simulink model "Maglev_Hardware_25a_R1"  (R2025a)
settings: Solver=FixedStepDiscrete  StartTime=0.0  StopTime=inf  FixedStep=Ts  RelTol=1e-3  EnableMultiTasking=on
values from neighbouring files (symbols this model uses):
  k = 2.9626e-4    (= 0.00029626)    [rhs.m]    (also in simulate.m = -162.15)
undefined symbols (not defined in the file or in its folder): dend, dspblkCoreblockFVToolHelper, gcbh, numd
libraries: arduinolib x6, simulink x1
settings Model: ModifiedByFormat=C. Gokcek  SimulationMode=external  SILPILModeSetting=veronly  ExtModeTrigDuration=2  Creator=C. Gokcek  LastModifiedBy=C. Gokcek
settings SolverCC: AlgebraicLoopSolver=TrustRegion
settings DataIOCC: LimitDataPoints=on  SaveFormat=Array  SaveOutput=off  SaveTime=off  ReturnWorkspaceOutputs=off
settings OptimizationCC: EnhancedBackFolding=on  PassReuseOutputArgsThreshold=0.0  MaxStackSize=64  OptimizeBlockOrder=speed  DifferentSizesBufferReuse=on  OptimizationCustomize=off
settings DebuggingCC: UnderspecifiedInitializationDetection=Classic  MergeDetectMultiDrivingBlocksExec=none  ParameterTunabilityLossMsg=error  UnconnectedInputMsg=warning  UnconnectedOutputMsg=warning  UnconnectedLineMsg=warning  StateNameClashWarn=warning  SFUnexpectedBacktrackingDiag=warning  SFNoUnconditionalDefaultTransitionDiag=warning  SFExecutionAtInitializationDiag=none  ArithmeticOperatorsInVariantConditions=warning
settings HardwareCC: ProdBitPerInt=16.0  ProdBitPerPointer=16.0  ProdBitPerSizeT=16.0  ProdBitPerPtrDiffT=16.0  ProdLargestAtomicFloat=None  ProdWordSize=8.0  ProdHWDeviceType=Atmel->AVR  UseEmbeddedCoderFeatures=off  UseSimulinkCoderFeatures=off
settings ModelReferenceCC: EnableRefExpFcnMdlSchedulingChecks=on  PropagateSignalLabelsOutOfModel=off
settings SFSimCC: SimUseLocalCustomCode=off  MATLABDynamicMemAlloc=off  CustomCodeUndefinedFunction=UseInterfaceOnly
settings RTWCC: SystemTargetFile=ert.tlc  HardwareBoard=Arduino Mega 2560  TemplateMakefile=ert_default_tmf  RTWVerbose=off  RTWUseLocalCustomCode=off  Toolchain=Arduino AVR  BuildConfiguration=Faster Runs  GPUComputeCapability=3.5  Description=Embedded Coder
settings CodeAppCC: ForceParamTrailComments=on  OperatorAnnotations=on  MangleLength=10.0
settings ERTTargetCC: ExtModeTransport=3.0  ExtModeStaticAllocSize=2048.0  InlinedParameterPlacement=Hierarchical  DynamicArrayContainerType=coder::array  ERTCustomFileBanners=off  SupportContinuousTime=on  SupportNonInlinedSFcns=on  RemoveResetFunc=off  SupportVariableSizeSignals=on  ModelStepFunctionPrototypeControlCompliant=off
settings ConfigComp: CovMetricSettings=dw  CovSaveCumulativeToWorkspaceVar=on  CovSaveSingleToWorkspaceVar=on  CovExternalEMLEnable=off

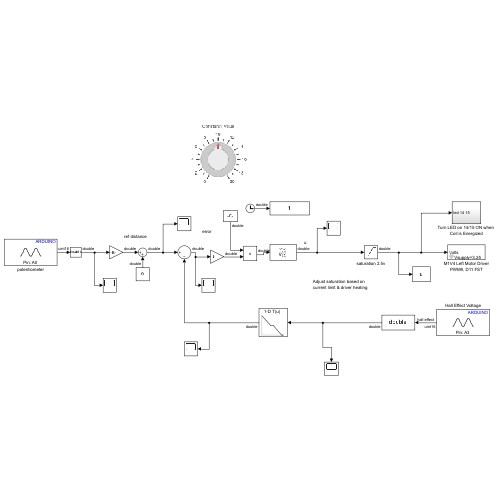
[thumbnail: Simulink's stored preview of the top-level diagram]
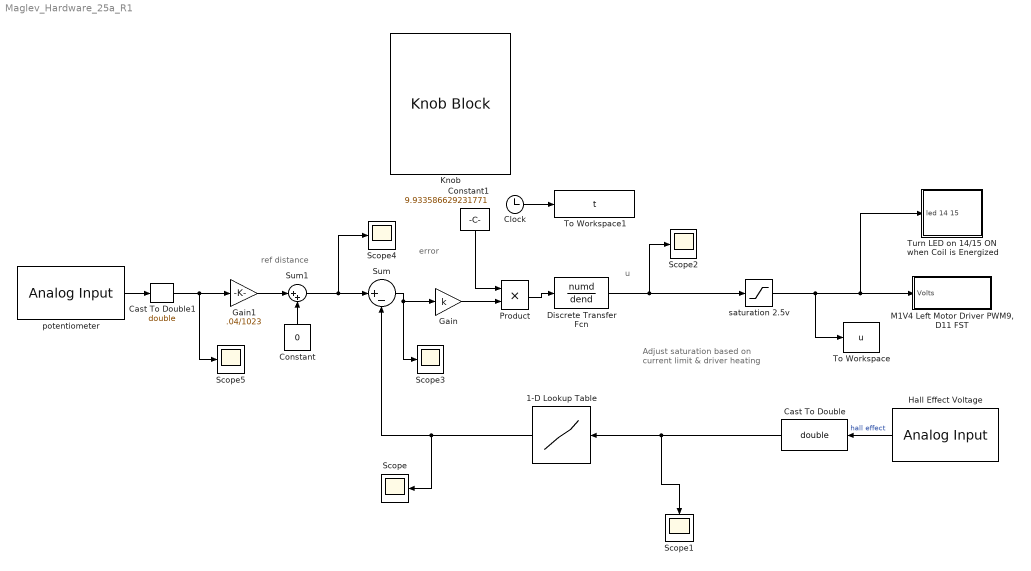
== system Maglev_Hardware_25a_R1 ==
  note: u
  note: error
  note: ref distance
  note: Adjust saturation based on
      | current limit & driver heating
  1-D Lookup Table : Lookup_n-D  NumberOfTableDimensions=1  BreakpointsForDimension1=[530;560;590;610;671;675;680;683]  Table=[0.038;0.034;0.03;0.03;0.022;0.022;0.022;0.022]  InternalRulePriority=Speed  RndMeth=Simplest
  Cast To Double : DataTypeConversion  OutDataTypeStr=double  SaturateOnIntegerOverflow=off  RndMeth=Floor
  Cast To Double1 : DataTypeConversion  OutDataTypeStr=double  SaturateOnIntegerOverflow=off  RndMeth=Floor
  Clock : Clock
  Constant : Constant  Value=0
  Constant1 : Constant  Value=9.933586629231771
  Discrete Transfer Fcn : DiscreteTransferFcn  LoadFcn=dspblkCoreblockFVToolHelper(gcbh,'load');  Numerator=numd  Denominator=dend
      settings: CopyFcn=dspblkCoreblockFVToolHelper(gcbh,'copy');  DeleteFcn=dspblkCoreblockFVToolHelper(gcbh,'close');  ModelCloseFcn=dspblkCoreblockFVToolHelper(gcbh,'close');  PreSaveFcn=dspblkCoreblockFVToolHelper(gcbh,'presave');  PostSaveFcn=dspblkCoreblockFVToolHelper(gcbh,'postsave');  CloseFcn=dspblkCoreblockFVToolHelper(gcbh,'close');
  Gain : Gain  Gain=k
  Gain1 : Gain  Gain=.04/1023
  Hall Effect Voltage : arduinolib/Analog Input  pinNumber=3  ReadResultsOnly=off  ConversionTriggerSource=Software  ExternalTriggerType=uint32( 0 )  OutputDataType=uint16  EnableConversionCompleteNotify=off  EnableOuputStatus=off  SampleTime=-1  blockPlatform=arduino
  Knob : KnobBlock  ScaleMax=20
  "M1V4 Left Motor Driver PWM9, D11 FST" : Subsystem  mask(Motor Driver){Vsupply=3.25}
      mask prompts: Vsupply "Driver Voltage"
      mask help:
      | Use a single PWM and a single Digtial out to control the magnitude and direction of a motor
      |
      | Specify driver supply voltage (3.25 for USB with SN754410)
      |
      | Driver supply voltage can be measured direcly by turning the motor fully on (100% duty cycle) and measuring the voltage across the motor leads.  This is the maximum voltage available to the motor and is used to scale from volts to PWM value 0-255.
      |
      | Note this value must be changed if the supply voltage to the driver is changed, for example, by using batteries.
      |
      | Vsupply is the maximum voltage your system is capable of supplying to system given the power supply. It needs to be measured depending on the power supply.
      mask Display:
      | port_label('input',1,'Volts')
      | text(15,5,['Vsupply=' num2str(Vsupply)])
  Product : Product
  Scope{,1..5} (6 alike) : Scope
      Scope settings: ActiveDisplayYMinimum=0.017726842779666189  ActiveDisplayYMaximum=0.11947479797527194
      Scope1 settings: ActiveDisplayYMinimum=999.02204895019531  ActiveDisplayYMaximum=1010.9426727294922
      Scope2 settings: ActiveDisplayYMinimum=-5.1897578239440918  ActiveDisplayYMaximum=11.745166301727295  DataLoggingVariableName=ScopeData2
      Scope3 settings: ActiveDisplayYMinimum=-0.0882034440588378  ActiveDisplayYMaximum=0.10637266834299446  DataLoggingVariableName=ScopeData3
      Scope4 settings: ActiveDisplayYMinimum=-0.00753435309113358  ActiveDisplayYMaximum=0.051082564719955821  DataLoggingVariableName=ScopeData4
      Scope5 settings: ActiveDisplayYMinimum=596.875  ActiveDisplayYMaximum=598.125  DataLoggingVariableName=ScopeData5
  Sum : Sum  Inputs=|+-
  Sum1 : Sum  Inputs=|++
  To Workspace : ToWorkspace  VariableName=u  SampleTime=-1
      settings: Save2DSignal=2-D array (concatenate along first dimension)
  To Workspace1 : ToWorkspace  VariableName=t  SampleTime=-1
      settings: Save2DSignal=2-D array (concatenate along first dimension)
  Turn LED on 14/15 ON when Coil is Energized : Subsystem
  potentiometer : arduinolib/Analog Input  pinNumber=0  ReadResultsOnly=off  ConversionTriggerSource=Software  ExternalTriggerType=uint32( 0 )  OutputDataType=uint16  EnableConversionCompleteNotify=off  EnableOuputStatus=off  SampleTime=-1  blockPlatform=arduino
  saturation 2.5v : Saturate  UpperLimit=3  LowerLimit=-3
  wires:
  Hall Effect Voltage/1 -> Cast To Double/1  "hall effect"
  Clock/1 -> To Workspace1/1
  Sum/1 -> Scope3/1, Gain/1
  potentiometer/1 -> Cast To Double1/1
  Sum1/1 -> Scope4/1, Sum/1
  Cast To Double1/1 -> Gain1/1, Scope5/1
  Gain1/1 -> Sum1/1
  Constant/1 -> Sum1/2
  Product/1 -> Discrete Transfer Fcn/1
  Gain/1 -> Product/2
  Constant1/1 -> Product/1
  Cast To Double/1 -> 1-D Lookup Table/1, Scope1/1
  saturation 2.5v/1 -> To Workspace/1, "M1V4 Left Motor Driver PWM9, D11 FST"/1(Volts), Turn LED on 14/15 ON when Coil is Energized/1(led 14 15)
  Discrete Transfer Fcn/1 -> saturation 2.5v/1, Scope2/1
  1-D Lookup Table/1 -> Sum/2, Scope/1

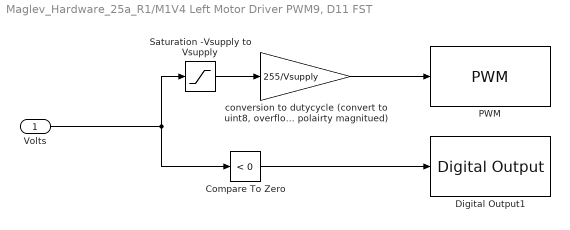
== system Maglev_Hardware_25a_R1/M1V4 Left Motor Driver PWM9, D11 FST ==
  Volts : Inport
  Compare To Zero : simulink/Logic and Bit Operations/Compare To Zero  relop=<  OutDataTypeStr=boolean
  Digital Output1 : arduinolib/Digital Output  pinNumber=11  Direction=output  blockPlatform=arduino
  PWM : arduinolib/PWM  pinNumber=9  frequencyType=Default  desiredFrequency=490.2  achievableFrequency=490.2
  Saturation -Vsupply to Vsupply : Saturate  UpperLimit=Vsupply  LowerLimit=-Vsupply  OutDataTypeStr=single
  "conversion to dutycycle (convert to uint8, overflow will provide reverse polairty magnitued)" : Gain  Gain=255/Vsupply  OutDataTypeStr=uint8
  wires:
  Volts/1 -> Compare To Zero/1, Saturation -Vsupply to Vsupply/1
  Saturation -Vsupply to Vsupply/1 -> "conversion to dutycycle (convert to uint8, overflow will provide reverse polairty magnitued)"/1
  "conversion to dutycycle (convert to uint8, overflow will provide reverse polairty magnitued)"/1 -> PWM/1
  Compare To Zero/1 -> Digital Output1/1

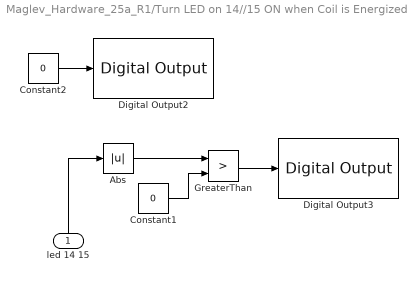
== system Maglev_Hardware_25a_R1/Turn LED on 14//15 ON when Coil is Energized ==
  led 14 15 : Inport
  Abs : Abs  SaturateOnIntegerOverflow=off
  Constant1 : Constant  Value=0  OutDataTypeStr=boolean  SampleTime=0
  Constant2 : Constant  Value=0  OutDataTypeStr=boolean  SampleTime=0
  Digital Output2 : arduinolib/Digital Output  pinNumber=14  Direction=output  blockPlatform=arduino
  Digital Output3 : arduinolib/Digital Output  pinNumber=15  Direction=output  blockPlatform=arduino
  GreaterThan : RelationalOperator  Operator=>  OutDataTypeStr=boolean  RndMeth=Simplest  InputSameDT=off
  wires:
  Constant2/1 -> Digital Output2/1
  led 14 15/1 -> Abs/1
  Abs/1 -> GreaterThan/1
  Constant1/1 -> GreaterThan/2
  GreaterThan/1 -> Digital Output3/1
